simulink model "qss_saab93_optigearOverload"  (Simulink 8.8)
settings: Solver=VariableStepDiscrete  StartTime=0.0  StopTime=1220  RelTol=1e-3  EnableMultiTasking=on
undefined symbols (not defined in the file or in its folder): g, h, rho
libraries: qss_tb_library x4
settings Model: Creator=Daniel  LastModifiedBy=grauers
settings OptimizationCC: ExpressionDepthLimit=2147483647  InitFltsAndDblsToZero=on
settings DebuggingCC: SaveWithParameterizedLinksMsg=none  SignalResolutionControl=TryResolveAllWithWarning  SolverPrmCheckMsg=warning  MultiTaskDSMMsg=warning  MultiTaskCondExecSysMsg=none  StrictBusMsg=None
settings GRTTargetCC: TargetFcnLib=ansi_tfl_tmw.mat

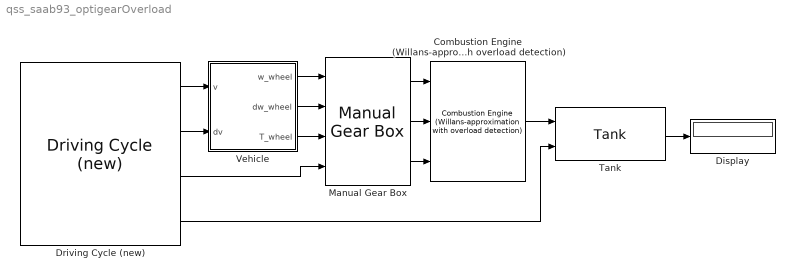
== system qss_saab93_optigearOverload ==
  Combustion Engine (Willans-approximation  with overload detection) : qss_tb_library/Energy Converter/Combustion Engine (Willans-approximation  with overload detection)  Tag=combustion engine  engine_type=Otto  V_d=1.985  theta_CE=0.05  S=78  B=90  maxTorque=[177 4300]  maxPower=[96 6100]  w_CE_upper=700  w_CE_idle=105  P_CE_idle=2600  P_aux=300  e=0.46  PI=2  p_me0g=1  ENABLE_FUEL_CUTOFF=on  T_CE_cutoff=5  P_CE_cutoff=0
  Display : Display
  Driving Cycle (new) : qss_tb_library/Driving Cycle/Driving Cycle (new)  Tag=cycle  cyclename1=NEDC  stepsize=1  autostop=on
  Manual Gear Box : qss_tb_library/Gear System/Manual Gear Box  Tag=transmission  i_1=first_gear  i_2=second_gear  i_3=third_gear  i_4=fourth_gear  i_5=fifth_gear  i_diff=diff_gear  e_GT=0.98  P_GT0=300  w_wheel_min=1
  Tank : qss_tb_library/Energy Source/Tank  Tag=tank  fuel=Gasoline  flag_cold_start=on
  Vehicle : Subsystem  Tag=vehicle  mask(Vehicle){m_f=1295+80+100, mt2m_f=5, A_f=2, d_wheel=0.62, cw=0.3, mu=0.013}
      mask prompts: m_f "Total mass of the vehicle [kg]"; mt2m_f "Rotating mass [%]"; A_f "Vehicle cross section [m^2]"; d_wheel "Wheel diameter [m]"; cw "Drag coefficient [-]"; mu "Rolling friction coefficient [-]"
      mask help:
      | This block computes the power required from the vehicle.
      |
      | Input:
      | =====
      | 	v		Speed [m/s]
      | 	dv		Acceleration [m/s^2]
      |
      | Output:
      | ======
      | 	w_wheel	Speed of the wheel [rad/s]
      | 	dw_wheel	Acceleration of the wheel [rad/s^2]
      | 	T_wheel	Torque on the wheel [Nm]
      mask init:
      | init_vehicle;
  wires:
  Vehicle/1(w_wheel) -> Manual Gear Box/1
  Vehicle/2(dw_wheel) -> Manual Gear Box/2
  Vehicle/3(T_wheel) -> Manual Gear Box/3
  Manual Gear Box/1 -> Combustion Engine (Willans-approximation  with overload detection)/1
  Manual Gear Box/2 -> Combustion Engine (Willans-approximation  with overload detection)/2
  Manual Gear Box/3 -> Combustion Engine (Willans-approximation  with overload detection)/3
  Combustion Engine (Willans-approximation  with overload detection)/1 -> Tank/1
  Driving Cycle (new)/3 -> Manual Gear Box/4
  Driving Cycle (new)/4 -> Tank/2
  Tank/1 -> Display/1
  Driving Cycle (new)/1 -> Vehicle/1(v)
  Driving Cycle (new)/2 -> Vehicle/2(dv)

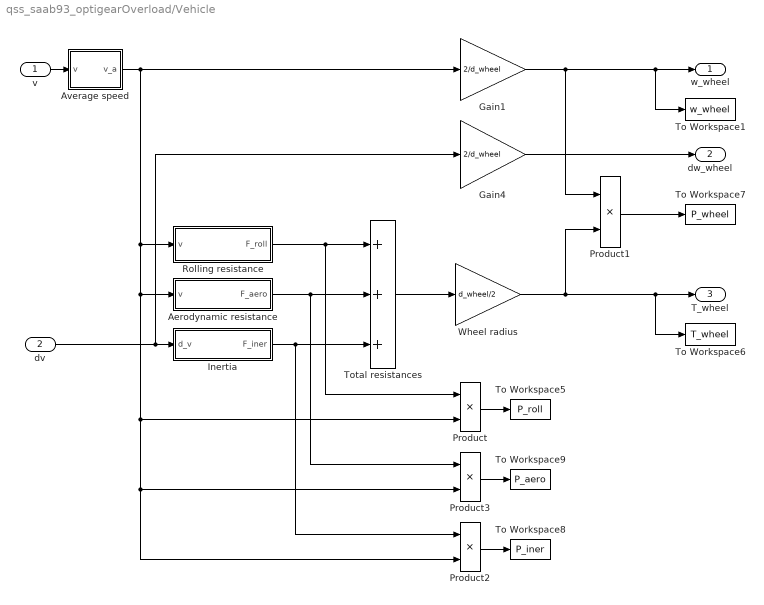
== system qss_saab93_optigearOverload/Vehicle ==
  v : Inport
  dv : Inport  Port=2
  Aerodynamic resistance : Subsystem
  Average speed : Subsystem
  Gain1 : Gain  Gain=2/d_wheel  SaturateOnIntegerOverflow=on  OutDataTypeStr=Inherit: Same as input  ParamDataTypeStr=Inherit: Same as input
  Gain4 : Gain  Gain=2/d_wheel  SaturateOnIntegerOverflow=on  OutDataTypeStr=Inherit: Same as input  ParamDataTypeStr=Inherit: Same as input
  Inertia : Subsystem
  Product{,1..3} (4 alike) : Product  SaturateOnIntegerOverflow=on  RndMeth=Zero  InputSameDT=on  OutDataTypeStr=Inherit: Same as first input
  Rolling resistance : Subsystem
  To Workspace1 : ToWorkspace  VariableName=w_wheel  SampleTime=-1
  To Workspace5 : ToWorkspace  VariableName=P_roll  SampleTime=-1
  To Workspace6 : ToWorkspace  VariableName=T_wheel  SampleTime=-1
  To Workspace7 : ToWorkspace  VariableName=P_wheel  SampleTime=-1
  To Workspace8 : ToWorkspace  VariableName=P_iner  SampleTime=-1
  To Workspace9 : ToWorkspace  VariableName=P_aero  SampleTime=-1
  Total resistances : Sum  Inputs=+++  SaturateOnIntegerOverflow=on  InputSameDT=on  OutDataTypeStr=Inherit: Same as first input
  Wheel radius : Gain  Gain=d_wheel/2  SaturateOnIntegerOverflow=on  OutDataTypeStr=Inherit: Same as input  ParamDataTypeStr=Inherit: Same as input
  w_wheel : Outport  InitialOutput=0
  dw_wheel : Outport  Port=2  InitialOutput=0
  T_wheel : Outport  Port=3  InitialOutput=0
  wires:
  Product/1 -> To Workspace5/1
  Product1/1 -> To Workspace7/1
  Product3/1 -> To Workspace9/1
  Product2/1 -> To Workspace8/1
  v/1 -> Average speed/1(v)
  dv/1 -> Gain4/1, Inertia/1(d_v)
  Average speed/1(v_a) -> Rolling resistance/1(v), Product2/2, Product3/2, Product/2, Aerodynamic resistance/1(v), Gain1/1
  Wheel radius/1 -> To Workspace6/1, T_wheel/1, Product1/2
  Total resistances/1 -> Wheel radius/1
  Inertia/1(F_iner) -> Product2/1, Total resistances/3
  Aerodynamic resistance/1(F_aero) -> Total resistances/2, Product3/1
  Rolling resistance/1(F_roll) -> Product/1, Total resistances/1
  Gain1/1 -> To Workspace1/1, w_wheel/1, Product1/1
  Gain4/1 -> dw_wheel/1

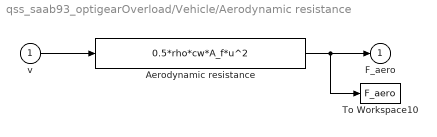
== system qss_saab93_optigearOverload/Vehicle/Aerodynamic resistance ==
  v : Inport
  Aerodynamic resistance : Fcn  Expr=0.5*rho*cw*A_f*u^2
  To Workspace10 : ToWorkspace  VariableName=F_aero  SampleTime=-1
  F_aero : Outport  InitialOutput=0
  wires:
  Aerodynamic resistance/1 -> To Workspace10/1, F_aero/1
  v/1 -> Aerodynamic resistance/1

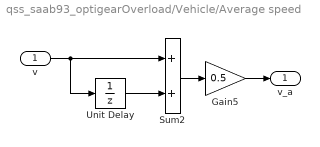
== system qss_saab93_optigearOverload/Vehicle/Average speed ==
  v : Inport
  Gain5 : Gain  Gain=0.5  SaturateOnIntegerOverflow=on  OutDataTypeStr=Inherit: Same as input  ParamDataTypeStr=Inherit: Same as input
  Sum2 : Sum  SaturateOnIntegerOverflow=on  InputSameDT=on  OutDataTypeStr=Inherit: Same as first input
  Unit Delay : UnitDelay  SampleTime=h
  v_a : Outport  InitialOutput=0
  wires:
  v/1 -> Unit Delay/1, Sum2/1
  Gain5/1 -> v_a/1
  Sum2/1 -> Gain5/1
  Unit Delay/1 -> Sum2/2

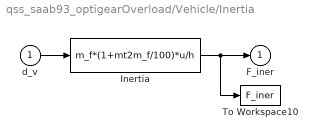
== system qss_saab93_optigearOverload/Vehicle/Inertia ==
  d_v : Inport
  Inertia : Fcn  Expr=m_f*(1+mt2m_f/100)*u/h
  To Workspace10 : ToWorkspace  VariableName=F_iner  SampleTime=-1
  F_iner : Outport  InitialOutput=0
  wires:
  d_v/1 -> Inertia/1
  Inertia/1 -> To Workspace10/1, F_iner/1

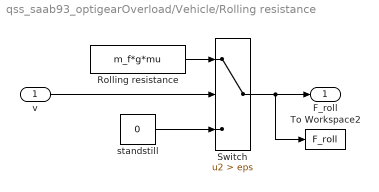
== system qss_saab93_optigearOverload/Vehicle/Rolling resistance ==
  v : Inport
  Rolling resistance : Constant  Value=m_f*g*mu
  Switch : Switch  Criteria=u2 > Threshold  Threshold=eps
  To Workspace2 : ToWorkspace  VariableName=F_roll  SampleTime=-1
  standstill : Constant  Value=0
  F_roll : Outport
  wires:
  Rolling resistance/1 -> Switch/1
  standstill/1 -> Switch/3
  v/1 -> Switch/2
  Switch/1 -> F_roll/1, To Workspace2/1
